simulink model "HeatRegulatorApp"  (R2015a)
settings: Solver=FixedStepDiscrete  StartTime=0.0  StopTime=10.0  RelTol=1e-3
undefined symbols (not defined in the file): Position, SeatHeatingControllerSetPosition
settings Model: Creator=Morya  LastModifiedBy=Morya
settings DataIOCC: SaveFormat=StructureWithTime
settings OptimizationCC: ZeroExternalMemoryAtStartup=off  ZeroInternalMemoryAtStartup=off  OptimizeModelRefInitCode=on  LifeSpan=1
settings ModelReferenceCC: ModelReferenceNumInstancesAllowed=Single
settings RTWCC: SystemTargetFile=autosar.tlc  GenCodeOnly=on  TemplateMakefile=ert_default_tmf  Description=AUTOSAR
settings CodeAppCC: IgnoreCustomStorageClasses=off
settings STFCustomTargetCC: GenerateSampleERTMain=off  ParMdlRefBuildCompliant=on  CompOptLevelCompliant=on  IncludeMdlTerminateFcn=off  CombineOutputUpdateFcns=on  SuppressErrorStatus=on  ERTFirstTimeCompliant=on  SupportNonFinite=off  SupportComplex=off  SupportContinuousTime=off  SupportVariableSizeSignals=off  AutosarCompliant=on  SystemTargetFile=autosar.tlc
settings ERTTargetCC: GenerateSampleERTMain=off  ParMdlRefBuildCompliant=on  CompOptLevelCompliant=on  IncludeMdlTerminateFcn=off  SuppressErrorStatus=on  ERTFirstTimeCompliant=on  SupportNonFinite=off  SupportComplex=off  SupportContinuousTime=off  SupportVariableSizeSignals=off  AutosarCompliant=on  ERTCustomFileTemplate=example_file_process.tlc

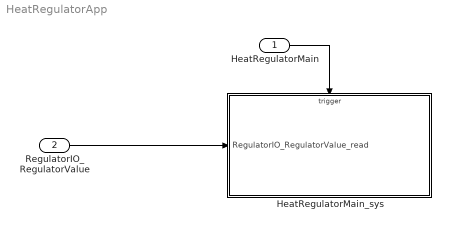
== system HeatRegulatorApp ==
  HeatRegulatorMain : Inport  OutputFunctionCall=on
  RegulatorIO_RegulatorValue : Inport  Port=2  OutDataTypeStr=Int32  PortDimensions=1
  HeatRegulatorMain_sys : Subsystem
  wires:
  HeatRegulatorMain/1 -> HeatRegulatorMain_sys/Trigger
  RegulatorIO_RegulatorValue/1 -> HeatRegulatorMain_sys/1(RegulatorIO_RegulatorValue_read)

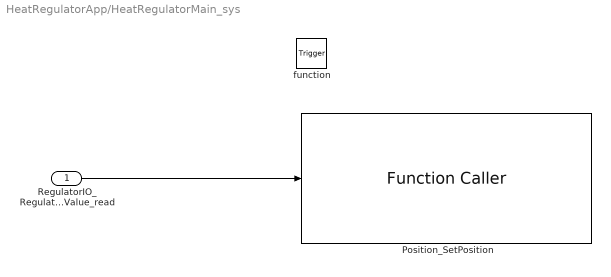
== system HeatRegulatorApp/HeatRegulatorMain_sys ==
  RegulatorIO_RegulatorValue_read : Inport
  function : TriggerPort  TriggerType=function-call
  Position_SetPosition : FunctionCaller  FunctionPrototype=SeatHeatingControllerSetPosition(Position)  InputArgumentSpecifications=P_Int32
  wires:
  RegulatorIO_RegulatorValue_read/1 -> Position_SetPosition/1
